simulink model "epc_4_4_1"  (R2023b)
settings: Solver=VariableStepAuto  StartTime=0.0  StopTime=10.0  MaxStep=0.01  RelTol=1e-3
settings Model: Creator=86186  LastModifiedBy=86186

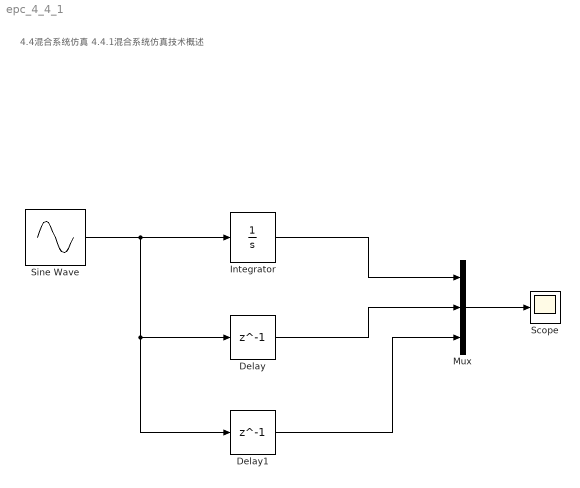
== system epc_4_4_1 ==
  note: 4.4混合系统仿真
      | 4.4.1混合系统仿真技术概述
  Delay : Delay  DelayLength=1  InitialCondition=0  SampleTime=0.5
  Delay1 : Delay  DelayLength=1  InitialCondition=0  SampleTime=1.2
  Integrator : Integrator
  Mux : Mux  Inputs=3
  Scope : Scope
  Sine Wave : Sin  SampleTime=0
  wires:
  Sine Wave/1 -> Delay1/1, Delay/1, Integrator/1
  Integrator/1 -> Mux/1
  Delay/1 -> Mux/2
  Delay1/1 -> Mux/3
  Mux/1 -> Scope/1
